simulink subsystem "robotMotionPlant"  (R2022b)
settings: Solver=VariableStepAuto  StartTime=0.0  StopTime=10.0  RelTol=1e-3
settings Model: Creator=Sahil Gaurkar  LastModifiedBy=Sahil Gaurkar

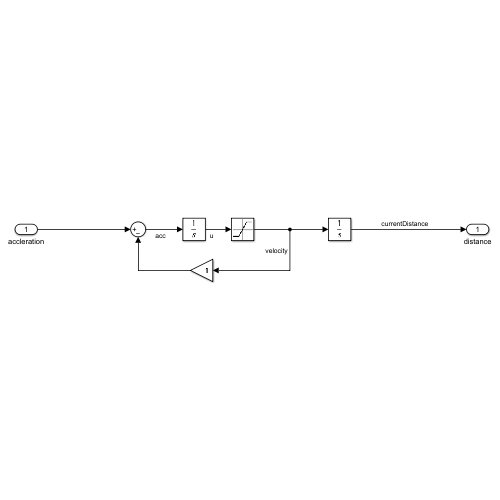
[thumbnail: Simulink's stored preview of the top-level diagram]
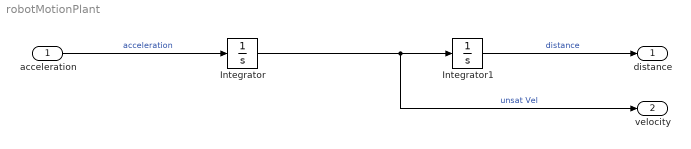
== system robotMotionPlant ==
  acceleration : Inport
  Integrator : Integrator  LimitOutput=on  UpperSaturationLimit=300  LowerSaturationLimit=0
  Integrator1 : Integrator
  distance : Outport
  velocity : Outport  Port=2
  wires:
  Integrator1/1 -> distance/1  "distance"
  acceleration/1 -> Integrator/1  "acceleration"
  Integrator/1 -> velocity/1, Integrator1/1  "unsat Vel"
